simulink model "FSAC2021_V1"  (R2014a)
settings: Solver=FixedStepDiscrete  StartTime=0.0  StopTime=inf  FixedStep=0.0005  RelTol=1e-3
model workspace (MAT data in the model file):
  MCOS : class17 (value not decoded)
  MCOS : class17 (value not decoded)
  MCOS : class17 (value not decoded)
  MCOS : class17 (value not decoded)
  MCOS : class17 (value not decoded)
  MCOS : class17 (value not decoded)
  MCOS : class17 (value not decoded)
  MCOS : class17 (value not decoded)
  MCOS : class17 (value not decoded)
  MCOS : class17 (value not decoded)
  MCOS : class17 (value not decoded)
  MCOS : class17 (value not decoded)
  MCOS : class17 (value not decoded)
  MCOS : class17 (value not decoded)
  MCOS : class17 (value not decoded)
  MCOS : class17 (value not decoded)
  MCOS : class17 (value not decoded)
  MCOS : class17 (value not decoded)
  MCOS : class17 (value not decoded)
  BUZZER_START = 1
  MCOS : class17 (value not decoded)
  MCOS : class17 (value not decoded)
  MCOS : class17 (value not decoded)
  MCOS : class17 (value not decoded)
  MCOS : class17 (value not decoded)
  MCOS : class17 (value not decoded)
  MCOS : class17 (value not decoded)
  MCOS : class17 (value not decoded)
  MCOS : class17 (value not decoded)
  MCOS : class17 (value not decoded)
  MCOS : class17 (value not decoded)
  MCOS : class17 (value not decoded)
  MCOS : class17 (value not decoded)
  MCOS : class17 (value not decoded)
  MCOS : class17 (value not decoded)
  MCOS : class17 (value not decoded)
  MCOS : class17 (value not decoded)
  MCOS : class17 (value not decoded)
  MCOS : class17 (value not decoded)
  MCOS : class17 (value not decoded)
  MCOS : class17 (value not decoded)
  MCOS : class17 (value not decoded)
  MCOS : class17 (value not decoded)
  MCOS : class17 (value not decoded)
  MCOS : class17 (value not decoded)
  MCOS : class17 (value not decoded)
  MCOS : class17 (value not decoded)
  MCOS : class17 (value not decoded)
  MCOS : class17 (value not decoded)
  MCOS : class17 (value not decoded)
  MCOS : class17 (value not decoded)
  MCOS : class17 (value not decoded)
  MCOS : class17 (value not decoded)
  MCOS : class17 (value not decoded)
  MCOS : class17 (value not decoded)
  MCOS : class17 (value not decoded)
  MCOS : class17 (value not decoded)
  MCOS : class17 (value not decoded)
  Brake = 11
  MCOS : class17 (value not decoded)
  MCOS : class17 (value not decoded)
  MCOS : class17 (value not decoded)
  MCOS : class17 (value not decoded)
  MCOS : class17 (value not decoded)
  MCOS : class17 (value not decoded)
  MCOS : class17 (value not decoded)
  MCOS : class17 (value not decoded)
  Sensor_Acc_b = 101.85
  Sensor_Acc_k = -0.0185
  Str_Sen_Orig_Angle = -341
  MCOS : class17 (value not decoded)
  Tire_D = 0.47
  T = 0.05
libraries: simulink x189, ec55xxlib x135
(part 6 of 9)

== system FSAC2021_V1/CAN_SEND/Subsystem1/MOTEC_ENCODER1/Str_Encoder6 ==
  Str_Encoder6 : Inport
  Str_Encoder6Ron : Rounding  Operator=round
  Str_Encoder6_1sat : Saturate  UpperLimit=255  LowerLimit=0
  Str_Encoder6_Convert : DataTypeConversion  OutDataTypeStr=uint8
  Str_Encoder6_Convert1 : DataTypeConversion  OutDataTypeStr=uint32
  Str_Encoder6_D : Product  Inputs=*/
  Str_Encoder6_F : Constant  OutDataTypeStr=single
  Str_Encoder6_L : simulink/Logic and Bit Operations/Bitwise Operator  logicop=AND  UseBitMask=on  BitMask=255  BitMaskRealWorld=Stored Integer
  Str_Encoder6_O : Constant  Value=0  OutDataTypeStr=single
  Str_Encoder6_S : ArithShift
  Str_Encoder6_sat : Saturate  UpperLimit=255  LowerLimit=0
  Str_Encoder6_st : Sum  Inputs=+-
  output6 : Outport
  wires:
  Str_Encoder6/1 -> Str_Encoder6_sat/1
  Str_Encoder6_sat/1 -> Str_Encoder6_st/1
  Str_Encoder6_O/1 -> Str_Encoder6_st/2
  Str_Encoder6_st/1 -> Str_Encoder6_D/1
  Str_Encoder6_F/1 -> Str_Encoder6_D/2
  Str_Encoder6_D/1 -> Str_Encoder6Ron/1
  Str_Encoder6Ron/1 -> Str_Encoder6_S/1
  Str_Encoder6_S/1 -> Str_Encoder6_1sat/1
  Str_Encoder6_1sat/1 -> Str_Encoder6_Convert1/1
  Str_Encoder6_Convert1/1 -> Str_Encoder6_L/1
  Str_Encoder6_L/1 -> Str_Encoder6_Convert/1
  Str_Encoder6_Convert/1 -> output6/1

== system FSAC2021_V1/CAN_SEND/Subsystem1/MOTEC_NMT/NMT_nodectrl ==
  NMT_nodectrl : Inport
  NMT_nodectrlRon : Rounding  Operator=round
  NMT_nodectrl_1sat : Saturate  UpperLimit=255  LowerLimit=0
  NMT_nodectrl_Convert : DataTypeConversion  OutDataTypeStr=uint8
  NMT_nodectrl_Convert1 : DataTypeConversion  OutDataTypeStr=uint32
  NMT_nodectrl_D : Product  Inputs=*/
  NMT_nodectrl_F : Constant  OutDataTypeStr=single
  NMT_nodectrl_L : simulink/Logic and Bit Operations/Bitwise Operator  logicop=AND  UseBitMask=on  BitMask=255  BitMaskRealWorld=Stored Integer
  NMT_nodectrl_O : Constant  Value=0  OutDataTypeStr=single
  NMT_nodectrl_S : ArithShift
  NMT_nodectrl_sat : Saturate  UpperLimit=255  LowerLimit=0
  NMT_nodectrl_st : Sum  Inputs=+-
  output2 : Outport
  wires:
  NMT_nodectrl/1 -> NMT_nodectrl_sat/1
  NMT_nodectrl_sat/1 -> NMT_nodectrl_st/1
  NMT_nodectrl_O/1 -> NMT_nodectrl_st/2
  NMT_nodectrl_st/1 -> NMT_nodectrl_D/1
  NMT_nodectrl_F/1 -> NMT_nodectrl_D/2
  NMT_nodectrl_D/1 -> NMT_nodectrlRon/1
  NMT_nodectrlRon/1 -> NMT_nodectrl_S/1
  NMT_nodectrl_S/1 -> NMT_nodectrl_1sat/1
  NMT_nodectrl_1sat/1 -> NMT_nodectrl_Convert1/1
  NMT_nodectrl_Convert1/1 -> NMT_nodectrl_L/1
  NMT_nodectrl_L/1 -> NMT_nodectrl_Convert/1
  NMT_nodectrl_Convert/1 -> output2/1

== system FSAC2021_V1/CAN_SEND/Subsystem1/MOTEC_NMT/NMT_nodeorder ==
  NMT_nodeorder : Inport
  NMT_nodeorderRon : Rounding  Operator=round
  NMT_nodeorder_1sat : Saturate  UpperLimit=255  LowerLimit=0
  NMT_nodeorder_Convert : DataTypeConversion  OutDataTypeStr=uint8
  NMT_nodeorder_Convert1 : DataTypeConversion  OutDataTypeStr=uint32
  NMT_nodeorder_D : Product  Inputs=*/
  NMT_nodeorder_F : Constant  OutDataTypeStr=single
  NMT_nodeorder_L : simulink/Logic and Bit Operations/Bitwise Operator  logicop=AND  UseBitMask=on  BitMask=255  BitMaskRealWorld=Stored Integer
  NMT_nodeorder_O : Constant  Value=0  OutDataTypeStr=single
  NMT_nodeorder_S : ArithShift
  NMT_nodeorder_sat : Saturate  UpperLimit=255  LowerLimit=0
  NMT_nodeorder_st : Sum  Inputs=+-
  output1 : Outport
  wires:
  NMT_nodeorder/1 -> NMT_nodeorder_sat/1
  NMT_nodeorder_sat/1 -> NMT_nodeorder_st/1
  NMT_nodeorder_O/1 -> NMT_nodeorder_st/2
  NMT_nodeorder_st/1 -> NMT_nodeorder_D/1
  NMT_nodeorder_F/1 -> NMT_nodeorder_D/2
  NMT_nodeorder_D/1 -> NMT_nodeorderRon/1
  NMT_nodeorderRon/1 -> NMT_nodeorder_S/1
  NMT_nodeorder_S/1 -> NMT_nodeorder_1sat/1
  NMT_nodeorder_1sat/1 -> NMT_nodeorder_Convert1/1
  NMT_nodeorder_Convert1/1 -> NMT_nodeorder_L/1
  NMT_nodeorder_L/1 -> NMT_nodeorder_Convert/1
  NMT_nodeorder_Convert/1 -> output1/1

== system FSAC2021_V1/CAN_SEND/Subsystem2/BCU_MTR_MOVE_AB/Brake_mtr_goalpos ==
  Brake_mtr_goalpos : Inport
  Brake_mtr_goalposABS : Abs
  Brake_mtr_goalposBitCov : DataTypeConversion  OutDataTypeStr=uint32
  Brake_mtr_goalposBitCov1 : DataTypeConversion  OutDataTypeStr=uint32
  Brake_mtr_goalposBitCov2 : DataTypeConversion  OutDataTypeStr=uint8
  Brake_mtr_goalposCOV : DataTypeConversion  OutDataTypeStr=uint8
  Brake_mtr_goalposCOV1 : DataTypeConversion  OutDataTypeStr=uint8
  Brake_mtr_goalposCOV2 : DataTypeConversion  OutDataTypeStr=uint8
  Brake_mtr_goalposCS : ArithShift  BitShiftNumber=-32
  Brake_mtr_goalposConS : Constant  OutDataTypeStr=single
  Brake_mtr_goalposCosR : Constant  Value=0  OutDataTypeStr=uint8
  Brake_mtr_goalposROP : RelationalOperator  Operator=<  OutDataTypeStr=boolean
  Brake_mtr_goalposRon : Rounding  Operator=round
  Brake_mtr_goalposSW : Switch  Criteria=u2 ~= 0
  Brake_mtr_goalpos_1sat : Saturate  UpperLimit=4294967295  LowerLimit=0
  Brake_mtr_goalpos_And : simulink/Logic and Bit Operations/Bitwise Operator  logicop=AND  UseBitMask=off  NumInputPorts=2  BitMask=bin2dec('11011001')  BitMaskRealWorld=Stored Integer
  Brake_mtr_goalpos_And1 : simulink/Logic and Bit Operations/Bitwise Operator  logicop=AND  UseBitMask=off  NumInputPorts=2  BitMask=bin2dec('11011001')  BitMaskRealWorld=Stored Integer
  Brake_mtr_goalpos_And1_C : Constant  Value=65535
  Brake_mtr_goalpos_And2 : simulink/Logic and Bit Operations/Bitwise Operator  logicop=AND  UseBitMask=off  NumInputPorts=2  BitMask=bin2dec('11011001')  BitMaskRealWorld=Stored Integer
  Brake_mtr_goalpos_And2_C : Constant  Value=255  OutDataTypeStr=uint32
  Brake_mtr_goalpos_And_C : Constant  Value=16777215
  Brake_mtr_goalpos_Convert : DataTypeConversion  OutDataTypeStr=uint32
  Brake_mtr_goalpos_D{,1..3} (4 alike) : Product  Inputs=*/
  Brake_mtr_goalpos_F : Constant  OutDataTypeStr=single
  Brake_mtr_goalpos_L : simulink/Logic and Bit Operations/Bitwise Operator  logicop=AND  UseBitMask=on  BitMask=4294967295  BitMaskRealWorld=Stored Integer
  Brake_mtr_goalpos_O : Constant  Value=0  OutDataTypeStr=single
  Brake_mtr_goalpos_S : ArithShift
  Brake_mtr_goalpos_sat : Saturate  UpperLimit=2147483647  LowerLimit=-2147483648
  Brake_mtr_goalpos_st : Sum  Inputs=+-
  Brake_mtr_goalpos_swtsig : Switch  Criteria=u2 ~= 0
  Brake_mtr_goalposoutput2_C : Constant  Value=256
  Brake_mtr_goalposoutput3_C : Constant  Value=65536
  Brake_mtr_goalposoutput4_C : Constant  Value=16777216
  Brake_mtr_goalpossatAbs : Saturate  UpperLimit=2147483647  LowerLimit=0
  Brake_mtr_goalpossubcon : Sum  Inputs=+-
  output1 : Outport
  output2 : Outport  Port=2
  output3 : Outport  Port=3
  output4 : Outport  Port=4
  wires:
  Brake_mtr_goalpos/1 -> Brake_mtr_goalpos_sat/1
  Brake_mtr_goalpos_sat/1 -> Brake_mtr_goalpos_st/1
  Brake_mtr_goalpos_O/1 -> Brake_mtr_goalpos_st/2
  Brake_mtr_goalpos_st/1 -> Brake_mtr_goalpos_D/1
  Brake_mtr_goalpos_F/1 -> Brake_mtr_goalpos_D/2
  Brake_mtr_goalpos_D/1 -> Brake_mtr_goalposRon/1
  Brake_mtr_goalpossatAbs/1 -> Brake_mtr_goalpos_swtsig/1, Brake_mtr_goalposSW/3
  Brake_mtr_goalposROP/1 -> Brake_mtr_goalpos_swtsig/2, Brake_mtr_goalposSW/2
  Brake_mtr_goalposRon/1 -> Brake_mtr_goalposROP/1, Brake_mtr_goalposABS/1, Brake_mtr_goalpos_swtsig/3
  Brake_mtr_goalpos_swtsig/1 -> Brake_mtr_goalpossubcon/2
  Brake_mtr_goalposCosR/1 -> Brake_mtr_goalposROP/2
  Brake_mtr_goalposConS/1 -> Brake_mtr_goalposCS/1
  Brake_mtr_goalposCS/1 -> Brake_mtr_goalpossubcon/1
  Brake_mtr_goalposABS/1 -> Brake_mtr_goalpossatAbs/1
  Brake_mtr_goalpossubcon/1 -> Brake_mtr_goalposSW/1
  Brake_mtr_goalposSW/1 -> Brake_mtr_goalpos_S/1
  Brake_mtr_goalpos_S/1 -> Brake_mtr_goalpos_1sat/1
  Brake_mtr_goalpos_1sat/1 -> Brake_mtr_goalpos_Convert/1
  Brake_mtr_goalpos_Convert/1 -> Brake_mtr_goalpos_L/1
  Brake_mtr_goalpos_L/1 -> Brake_mtr_goalpos_And1/1, Brake_mtr_goalpos_And2/1, Brake_mtr_goalpos_And/1, Brake_mtr_goalpos_D1/1
  Brake_mtr_goalposoutput4_C/1 -> Brake_mtr_goalpos_D1/2
  Brake_mtr_goalpos_D1/1 -> Brake_mtr_goalposCOV/1
  Brake_mtr_goalposCOV/1 -> output1/1
  Brake_mtr_goalpos_And_C/1 -> Brake_mtr_goalposBitCov/1
  Brake_mtr_goalposBitCov/1 -> Brake_mtr_goalpos_And/2
  Brake_mtr_goalpos_And/1 -> Brake_mtr_goalpos_D2/1
  Brake_mtr_goalposoutput3_C/1 -> Brake_mtr_goalpos_D2/2
  Brake_mtr_goalpos_D2/1 -> Brake_mtr_goalposCOV1/1
  Brake_mtr_goalposCOV1/1 -> output2/1
  Brake_mtr_goalpos_And1_C/1 -> Brake_mtr_goalposBitCov1/1
  Brake_mtr_goalposBitCov1/1 -> Brake_mtr_goalpos_And1/2
  Brake_mtr_goalpos_And1/1 -> Brake_mtr_goalpos_D3/1
  Brake_mtr_goalposoutput2_C/1 -> Brake_mtr_goalpos_D3/2
  Brake_mtr_goalpos_D3/1 -> Brake_mtr_goalposCOV2/1
  Brake_mtr_goalposCOV2/1 -> output3/1
  Brake_mtr_goalpos_And2_C/1 -> Brake_mtr_goalpos_And2/2
  Brake_mtr_goalpos_And2/1 -> Brake_mtr_goalposBitCov2/1
  Brake_mtr_goalposBitCov2/1 -> output4/1

== system FSAC2021_V1/CAN_SEND/Subsystem2/MOTOR_SPEED_CONTROL/Drive_Speed_Control ==
  Drive_Speed_Control : Inport
  BitCov : DataTypeConversion  OutDataTypeStr=uint8
  Drive_Speed_ControlCOV : DataTypeConversion  OutDataTypeStr=uint8
  Drive_Speed_ControlRon : Rounding  Operator=round
  Drive_Speed_Control_1sat : Saturate  UpperLimit=65535  LowerLimit=0
  Drive_Speed_Control_And : simulink/Logic and Bit Operations/Bitwise Operator  logicop=AND  UseBitMask=off  NumInputPorts=2  BitMask=bin2dec('11011001')  BitMaskRealWorld=Stored Integer
  Drive_Speed_Control_And_C : Constant  Value=255  OutDataTypeStr=uint32
  Drive_Speed_Control_Convert : DataTypeConversion  OutDataTypeStr=uint32
  Drive_Speed_Control_D : Product  Inputs=*/
  Drive_Speed_Control_D1 : Product  Inputs=*/
  Drive_Speed_Control_F : Constant  OutDataTypeStr=single
  Drive_Speed_Control_L : simulink/Logic and Bit Operations/Bitwise Operator  logicop=AND  UseBitMask=on  BitMask=65535  BitMaskRealWorld=Stored Integer
  Drive_Speed_Control_O : Constant  Value=0  OutDataTypeStr=single
  Drive_Speed_Control_S : ArithShift
  Drive_Speed_Control_sat : Saturate  UpperLimit=1500  LowerLimit=0
  Drive_Speed_Control_st : Sum  Inputs=+-
  Drive_Speed_Controloutput2_C : Constant  Value=256
  output1 : Outport
  output2 : Outport  Port=2
  wires:
  Drive_Speed_Control/1 -> Drive_Speed_Control_sat/1
  Drive_Speed_Control_sat/1 -> Drive_Speed_Control_st/1
  Drive_Speed_Control_O/1 -> Drive_Speed_Control_st/2
  Drive_Speed_Control_st/1 -> Drive_Speed_Control_D/1
  Drive_Speed_Control_F/1 -> Drive_Speed_Control_D/2
  Drive_Speed_Control_D/1 -> Drive_Speed_ControlRon/1
  Drive_Speed_ControlRon/1 -> Drive_Speed_Control_S/1
  Drive_Speed_Control_S/1 -> Drive_Speed_Control_1sat/1
  Drive_Speed_Control_1sat/1 -> Drive_Speed_Control_Convert/1
  Drive_Speed_Control_Convert/1 -> Drive_Speed_Control_L/1
  Drive_Speed_Control_L/1 -> Drive_Speed_Control_D1/1, Drive_Speed_Control_And/1
  Drive_Speed_Controloutput2_C/1 -> Drive_Speed_Control_D1/2
  Drive_Speed_Control_D1/1 -> Drive_Speed_ControlCOV/1
  Drive_Speed_ControlCOV/1 -> output2/1
  Drive_Speed_Control_And_C/1 -> Drive_Speed_Control_And/2
  Drive_Speed_Control_And/1 -> BitCov/1
  BitCov/1 -> output1/1

== system FSAC2021_V1/CAN_SEND/Subsystem3/BCU_STATUS_READ/status_reg_addr_start ==
  status_reg_addr_start : Inport
  status_reg_addr_startRon : Rounding  Operator=round
  status_reg_addr_start_1sat : Saturate  UpperLimit=255  LowerLimit=0
  status_reg_addr_start_Convert : DataTypeConversion  OutDataTypeStr=uint8
  status_reg_addr_start_Convert1 : DataTypeConversion  OutDataTypeStr=uint32
  status_reg_addr_start_D : Product  Inputs=*/
  status_reg_addr_start_F : Constant  OutDataTypeStr=single
  status_reg_addr_start_L : simulink/Logic and Bit Operations/Bitwise Operator  logicop=AND  UseBitMask=on  BitMask=255  BitMaskRealWorld=Stored Integer
  status_reg_addr_start_O : Constant  Value=0  OutDataTypeStr=single
  status_reg_addr_start_S : ArithShift
  status_reg_addr_start_sat : Saturate  UpperLimit=255  LowerLimit=0
  status_reg_addr_start_st : Sum  Inputs=+-
  output1 : Outport
  wires:
  status_reg_addr_start/1 -> status_reg_addr_start_sat/1
  status_reg_addr_start_sat/1 -> status_reg_addr_start_st/1
  status_reg_addr_start_O/1 -> status_reg_addr_start_st/2
  status_reg_addr_start_st/1 -> status_reg_addr_start_D/1
  status_reg_addr_start_F/1 -> status_reg_addr_start_D/2
  status_reg_addr_start_D/1 -> status_reg_addr_startRon/1
  status_reg_addr_startRon/1 -> status_reg_addr_start_S/1
  status_reg_addr_start_S/1 -> status_reg_addr_start_1sat/1
  status_reg_addr_start_1sat/1 -> status_reg_addr_start_Convert1/1
  status_reg_addr_start_Convert1/1 -> status_reg_addr_start_L/1
  status_reg_addr_start_L/1 -> status_reg_addr_start_Convert/1
  status_reg_addr_start_Convert/1 -> output1/1

== system FSAC2021_V1/CAN_SEND/Subsystem3/BCU_STATUS_READ/status_reg_num ==
  status_reg_num : Inport
  status_reg_numRon : Rounding  Operator=round
  status_reg_num_1sat : Saturate  UpperLimit=255  LowerLimit=0
  status_reg_num_Convert : DataTypeConversion  OutDataTypeStr=uint8
  status_reg_num_Convert1 : DataTypeConversion  OutDataTypeStr=uint32
  status_reg_num_D : Product  Inputs=*/
  status_reg_num_F : Constant  OutDataTypeStr=single
  status_reg_num_L : simulink/Logic and Bit Operations/Bitwise Operator  logicop=AND  UseBitMask=on  BitMask=255  BitMaskRealWorld=Stored Integer
  status_reg_num_O : Constant  Value=0  OutDataTypeStr=single
  status_reg_num_S : ArithShift
  status_reg_num_sat : Saturate  UpperLimit=255  LowerLimit=0
  status_reg_num_st : Sum  Inputs=+-
  output2 : Outport
  wires:
  status_reg_num/1 -> status_reg_num_sat/1
  status_reg_num_sat/1 -> status_reg_num_st/1
  status_reg_num_O/1 -> status_reg_num_st/2
  status_reg_num_st/1 -> status_reg_num_D/1
  status_reg_num_F/1 -> status_reg_num_D/2
  status_reg_num_D/1 -> status_reg_numRon/1
  status_reg_numRon/1 -> status_reg_num_S/1
  status_reg_num_S/1 -> status_reg_num_1sat/1
  status_reg_num_1sat/1 -> status_reg_num_Convert1/1
  status_reg_num_Convert1/1 -> status_reg_num_L/1
  status_reg_num_L/1 -> status_reg_num_Convert/1
  status_reg_num_Convert/1 -> output2/1

== system FSAC2021_V1/Controller/200ms_Duty/Light_Subsystem/BLINK  ==
  Action Port : ActionPort  ActionType=else
  Data Type Conversion : DataTypeConversion  OutDataTypeStr=uint8
  Logical Operator : Logic  Operator=NOT  AllPortsSameDT=off  OutDataTypeStr=boolean
  Unit Delay : UnitDelay  SampleTime=-1
  Out1 : Outport
  wires:
  Logical Operator/1 -> Data Type Conversion/1
  Data Type Conversion/1 -> Unit Delay/1, Out1/1
  Unit Delay/1 -> Logical Operator/1

== system FSAC2021_V1/Controller/200ms_Duty/Light_Subsystem/OFF ==
  Action Port : ActionPort  ActionType=elseif
  Constant : Constant  OutDataTypeStr=uint8
  Out1 : Outport
  wires:
  Constant/1 -> Out1/1

== system FSAC2021_V1/Controller/200ms_Duty/Light_Subsystem/ON ==
  Action Port : ActionPort  ActionType=then
  Constant : Constant  Value=0  OutDataTypeStr=uint8
  Out1 : Outport
  wires:
  Constant/1 -> Out1/1

== system FSAC2021_V1/Controller/200ms_Duty/Light_Subsystem1/BLINK ==
  Action Port : ActionPort  ActionType=else
  Data Type Conversion : DataTypeConversion  OutDataTypeStr=uint8
  Logical Operator : Logic  Operator=NOT  AllPortsSameDT=off  OutDataTypeStr=boolean
  Unit Delay : UnitDelay  SampleTime=-1
  Out1 : Outport
  wires:
  Unit Delay/1 -> Logical Operator/1
  Data Type Conversion/1 -> Out1/1, Unit Delay/1
  Logical Operator/1 -> Data Type Conversion/1

== system FSAC2021_V1/Controller/200ms_Duty/Light_Subsystem1/OFF ==
  Action Port : ActionPort  ActionType=elseif
  Constant : Constant  OutDataTypeStr=uint8
  Out1 : Outport
  wires:
  Constant/1 -> Out1/1

== system FSAC2021_V1/Controller/200ms_Duty/Light_Subsystem1/ON ==
  Action Port : ActionPort  ActionType=then
  Constant : Constant  Value=0  OutDataTypeStr=uint8
  Out1 : Outport
  wires:
  Constant/1 -> Out1/1

== system FSAC2021_V1/Controller/200ms_Duty/Light_Subsystem2/EBS_Horn ==
  Action Port : ActionPort  ActionType=else
  Chart : Stateflow chart  TreatAsAtomicUnit=on
  Buzzer_Pin : Outport
  Buzzer_Overflag : Outport  Port=2
  wires:
  Chart/1(Buzzer_Pin) -> Buzzer_Pin/1
  Chart/2(Buzzer_Overflag) -> Buzzer_Overflag/1

== system FSAC2021_V1/Controller/200ms_Duty/Light_Subsystem2/Start_Horn ==
  Action Port : ActionPort  ActionType=elseif
  Chart : Stateflow chart  TreatAsAtomicUnit=on
  Out1 : Outport
  wires:
  Chart/1(Buzzer_Pin) -> Out1/1

== system FSAC2021_V1/Controller/200ms_Duty/Light_Subsystem2/off ==
  Action Port : ActionPort  ActionType=then
  Constant : Constant  Value=0  OutDataTypeStr=uint8
  Out1 : Outport
  wires:
  Constant/1 -> Out1/1

== system FSAC2021_V1/Controller/50ms_Duty/Subsystem/Subsystem ==
  acc : Inport
  Acc_Flag : Inport  Port=2
  Enable : EnablePort
  Constant : Constant  Value=0
  Switch : Switch  Criteria=u2 > Threshold
  Acc_Cmd : Outport
  wires:
  Acc_Flag/1 -> Switch/2
  Constant/1 -> Switch/1
  acc/1 -> Switch/3
  Switch/1 -> Acc_Cmd/1

== system FSAC2021_V1/Controller/50ms_Duty/Subsystem/Subsystem1 ==
  IPC_Acc_Cmd : Inport
  IPC_Brk_Cmd : Inport  Port=2
  IPC_Str_Cmd : Inport  Port=3
  Enable : EnablePort
  Data Type Conversion : DataTypeConversion
  Gain : Gain  Gain=15
  Gain1 : Gain  Gain=0.134
  Saturation : Saturate  UpperLimit=13.4  LowerLimit=0
  Brk_Cmd : Outport
  Str_Cmd : Outport  Port=2
  Acc_Cmd : Outport  Port=3
  wires:
  IPC_Str_Cmd/1 -> Str_Cmd/1
  Gain/1 -> Acc_Cmd/1
  IPC_Brk_Cmd/1 -> Gain1/1
  Gain1/1 -> Saturation/1
  Saturation/1 -> Data Type Conversion/1
  IPC_Acc_Cmd/1 -> Gain/1
  Data Type Conversion/1 -> Brk_Cmd/1

== system FSAC2021_V1/Controller/50ms_Duty/Subsystem/Subsystem2 ==
  Enable : EnablePort
  Chart : Stateflow chart  TreatAsAtomicUnit=on
  ACC : Outport
  SteerCmd : Outport  Port=2
  Mission_Flag : Outport  Port=3
  wires:
  Chart/1(Mission_Flag) -> Mission_Flag/1
  Chart/3(ACC) -> ACC/1
  Chart/2(SteerCmd) -> SteerCmd/1

== system FSAC2021_V1/Controller/BCU_Controller/Brk_Move/Enabled Subsystem ==
  Enable : EnablePort
  Angle2Pulses : Subsystem  TreatAsAtomicUnit=on
  Constant : Constant  Value=BRK_Engaged_Angle  OutDataTypeStr=int8
  Engaged_Pulses : Outport
  Engaged_Angle : Outport  Port=2
  wires:
  Angle2Pulses/1(Pulses) -> Engaged_Pulses/1
  Constant/1 -> Angle2Pulses/1(Angle), Engaged_Angle/1

== system FSAC2021_V1/Controller/BCU_Controller/Brk_Move/Enabled Subsystem1 ==
  Engaged_Angle : Inport
  Enable : EnablePort
  Angle2Pulses : Subsystem  TreatAsAtomicUnit=on
  Gain : Gain  ParamDataTypeStr=int8  OutDataTypeStr=int8
  ToZero_Pulses : Outport
  wires:
  Angle2Pulses/1(Pulses) -> ToZero_Pulses/1
  Engaged_Angle/1 -> Gain/1
  Gain/1 -> Angle2Pulses/1(Angle)

== system FSAC2021_V1/Controller/BCU_Controller/Brk_Move/Enabled Subsystem2 ==
  note: 制动百分比
  note: 电机反转
  Brk_Prop : Inport
  Enable : EnablePort
  Angle2Pulses : Subsystem  TreatAsAtomicUnit=on
  Brk_Prop2Angle : Gain  Gain=Brk_Prop2Angle
  Gain : Gain  Gain=-1  ParamDataTypeStr=int8  OutDataTypeStr=single
  Move_Pulses : Outport
  wires:
  Gain/1 -> Angle2Pulses/1(Angle)
  Brk_Prop/1 -> Brk_Prop2Angle/1
  Brk_Prop2Angle/1 -> Gain/1
  Angle2Pulses/1(Pulses) -> Move_Pulses/1

== system FSAC2021_V1/DIAG/DIAG/ACC/Enabled Subsystem ==
  liquid_presuress : Inport
  Acc_Ctrl : Inport  Port=2
  Enable : EnablePort
  Chart : Stateflow chart  TreatAsAtomicUnit=on
  Acc_Flag : Outport
  wires:
  liquid_presuress/1 -> Chart/1(liquid_presuress)
  Acc_Ctrl/1 -> Chart/2(Acc)
  Chart/1(Acc_Flag) -> Acc_Flag/1

== system FSAC2021_V1/DIAG/DIAG/CAN_NODE_LOSTCOM/B_M_S_Check ==
  Brake_Node : Inport
  Motec_Node : Inport  Port=2
  RES_Node : Inport  Port=3
  Enable : EnablePort
  Chart : Stateflow chart  TreatAsAtomicUnit=on
      settings: RTWSystemCode=Reusable function
  Chart1 : Stateflow chart  TreatAsAtomicUnit=on
      settings: RTWSystemCode=Reusable function
  Logical Operator : Logic  AllPortsSameDT=off  OutDataTypeStr=boolean
  MeaModule1 : ec55xxlib/RapidECU_U2/11Calibration/MeaModule  signal=BRAKE
  MeaModule2 : ec55xxlib/RapidECU_U2/11Calibration/MeaModule  signal=MOTEC
  Node_Lost_Flag : Outport
  wires:
  Logical Operator/1 -> Node_Lost_Flag/1
  Brake_Node/1 -> Chart1/1(Input)
  MeaModule1/1 -> Logical Operator/1
  MeaModule2/1 -> Logical Operator/2
  Motec_Node/1 -> Chart/1(Input)
  Chart/1(Output) -> MeaModule2/1
  Chart1/1(Output) -> MeaModule1/1

== system FSAC2021_V1/DIAG/DIAG/CAN_NODE_LOSTCOM/Subsystem ==
  Motor_Node : Inport
  Enable : EnablePort
  Chart4 : Stateflow chart  TreatAsAtomicUnit=on
      settings: RTWSystemCode=Reusable function
  MeaModule1 : ec55xxlib/RapidECU_U2/11Calibration/MeaModule  signal=motor
  Node_Lost_Flag : Outport
  wires:
  MeaModule1/1 -> Node_Lost_Flag/1
  Motor_Node/1 -> Chart4/1(Input)
  Chart4/1(Output) -> MeaModule1/1

== system FSAC2021_V1/DIAG/DIAG/CAN_NODE_LOSTCOM/Subsystem1 ==
  StrSr_Node : Inport
  BMS_Node : Inport  Port=2
  AMI_Node : Inport  Port=3
  Chart2 : Stateflow chart  TreatAsAtomicUnit=on
      settings: RTWSystemCode=Reusable function
  Chart3 : Stateflow chart  TreatAsAtomicUnit=on
      settings: RTWSystemCode=Reusable function
  Chart4 : Stateflow chart  TreatAsAtomicUnit=on
      settings: RTWSystemCode=Reusable function
  Logical Operator : Logic  Inputs=3  AllPortsSameDT=off  OutDataTypeStr=boolean
  MeaModule3 : ec55xxlib/RapidECU_U2/11Calibration/MeaModule  signal=STRSNR
  MeaModule4 : ec55xxlib/RapidECU_U2/11Calibration/MeaModule  signal=BMS
  MeaModule5 : ec55xxlib/RapidECU_U2/11Calibration/MeaModule  signal=AMI_NODE
  Out1 : Outport
  wires:
  StrSr_Node/1 -> Chart2/1(Input)
  Chart2/1(Output) -> MeaModule3/1
  Chart4/1(Output) -> MeaModule5/1
  Chart3/1(Output) -> MeaModule4/1
  BMS_Node/1 -> Chart3/1(Input)
  AMI_Node/1 -> Chart4/1(Input)
  MeaModule3/1 -> Logical Operator/1
  MeaModule4/1 -> Logical Operator/2
  MeaModule5/1 -> Logical Operator/3
  Logical Operator/1 -> Out1/1

== system FSAC2021_V1/DIAG/DIAG/Res_Diag/Subsystem ==
  RES_SINGNAL : Inport
  Enable : EnablePort
  Chart1 : Stateflow chart  TreatAsAtomicUnit=on
      settings: RTWSystemCode=Reusable function
  Compare To Constant1 : simulink/Logic and Bit Operations/Compare To Constant  relop===  const=8  OutDataTypeStr=boolean
  Compare To Constant2 : simulink/Logic and Bit Operations/Compare To Constant  relop===  const=0  OutDataTypeStr=boolean
  Data Type Conversion1 : DataTypeConversion
  Data Type Conversion22 : DataTypeConversion
  Data Type Conversion23 : DataTypeConversion
  MeaModule1 : ec55xxlib/RapidECU_U2/11Calibration/MeaModule  signal=res_ebs_value
  RES_GO : Outport
  RES_EBS : Outport  Port=2
  wires:
  Compare To Constant1/1 -> Data Type Conversion22/1
  Data Type Conversion22/1 -> RES_GO/1
  Data Type Conversion23/1 -> MeaModule1/1
  RES_SINGNAL/1 -> Compare To Constant2/1, Compare To Constant1/1
  MeaModule1/1 -> RES_EBS/1
  Chart1/1(Output) -> Data Type Conversion23/1
  Compare To Constant2/1 -> Data Type Conversion1/1
  Data Type Conversion1/1 -> Chart1/1(Input)

== system FSAC2021_V1/DIAG/DIAG/TS_Diag/Subsystem ==
  Compare_Volt_mv : Inport
  Enable : EnablePort
  Compare To Constant3 : simulink/Logic and Bit Operations/Compare To Constant  relop=<  const=2  OutDataTypeStr=boolean
  TS_Error : Outport
  wires:
  Compare_Volt_mv/1 -> Compare To Constant3/1
  Compare To Constant3/1 -> TS_Error/1

== system FSAC2021_V1/DIAG/DIAG/TS_Diag/Subsystem1 ==
  Compare_Volt_mv : Inport
  Enable : EnablePort
  Compare To Constant3 : simulink/Logic and Bit Operations/Compare To Constant  relop=<  const=2  OutDataTypeStr=boolean
  TS_Error : Outport
  wires:
  Compare_Volt_mv/1 -> Compare To Constant3/1
  Compare To Constant3/1 -> TS_Error/1

== system FSAC2021_V1/DIAG/DIAG/TS_Diag/Subsystem2 ==
  Compare_Volt_mv : Inport
  Enable : EnablePort
  Compare To Constant3 : simulink/Logic and Bit Operations/Compare To Constant  relop=<  const=2  OutDataTypeStr=boolean
  TS_Error : Outport
  wires:
  Compare_Volt_mv/1 -> Compare To Constant3/1
  Compare To Constant3/1 -> TS_Error/1

== system FSAC2021_V1/Input_Process/KL_Sig_Process/Whl_Spd_Process/LPF ==
  note: y(t) = K*u(t) + (1-K)*y(t-1) = y(t-1) + K*[u(t)-y(t-1)]
      | 其中，K=dT/T，K一般介于0~1之间，dT是运行步长，T是时间常数；u是输入信号；y是输出信号。
  Filter : Inport
  Add : Sum  Inputs=+-  AccumDataTypeStr=single
  Add1 : Sum  AccumDataTypeStr=single
  Constant : Constant  Value=Filter_Factor
  Product : Product  OutDataTypeStr=single
  Unit Delay : UnitDelay  InitialCondition=1  SampleTime=-1
  Filtered : Outport
  wires:
  Add1/1 -> Unit Delay/1, Filtered/1
  Filter/1 -> Add/1
  Unit Delay/1 -> Add1/2, Add/2
  Add/1 -> Product/2
  Constant/1 -> Product/1
  Product/1 -> Add1/1

== system FSAC2021_V1/Input_Process/KL_Sig_Process/Whl_Spd_Process/LPF1 ==
  note: y(t) = K*u(t) + (1-K)*y(t-1) = y(t-1) + K*[u(t)-y(t-1)]
      | 其中，K=dT/T，K一般介于0~1之间，dT是运行步长，T是时间常数；u是输入信号；y是输出信号。
  Filter : Inport
  Add : Sum  Inputs=+-  AccumDataTypeStr=single
  Add1 : Sum  AccumDataTypeStr=single
  Constant : Constant  Value=Filter_Factor
  Product : Product  OutDataTypeStr=single
  Unit Delay : UnitDelay  InitialCondition=1  SampleTime=-1
  Filtered : Outport
  wires:
  Product/1 -> Add1/1
  Constant/1 -> Product/1
  Add/1 -> Product/2
  Unit Delay/1 -> Add/2, Add1/2
  Filter/1 -> Add/1
  Add1/1 -> Filtered/1, Unit Delay/1

== system FSAC2021_V1/Input_Process/KL_Sig_Process/Whl_Spd_Process/LPF2 ==
  note: y(t) = K*u(t) + (1-K)*y(t-1) = y(t-1) + K*[u(t)-y(t-1)]
      | 其中，K=dT/T，K一般介于0~1之间，dT是运行步长，T是时间常数；u是输入信号；y是输出信号。
  Filter : Inport
  Add : Sum  Inputs=+-  AccumDataTypeStr=single
  Add1 : Sum  AccumDataTypeStr=single
  Constant : Constant  Value=Filter_Factor
  Product : Product  OutDataTypeStr=single
  Unit Delay : UnitDelay  InitialCondition=1  SampleTime=-1
  Filtered : Outport
  wires:
  Add1/1 -> Unit Delay/1, Filtered/1
  Filter/1 -> Add/1
  Unit Delay/1 -> Add1/2, Add/2
  Add/1 -> Product/2
  Constant/1 -> Product/1
  Product/1 -> Add1/1

== system FSAC2021_V1/Input_Process/KL_Sig_Process/Whl_Spd_Process/LPF3 ==
  note: y(t) = K*u(t) + (1-K)*y(t-1) = y(t-1) + K*[u(t)-y(t-1)]
      | 其中，K=dT/T，K一般介于0~1之间，dT是运行步长，T是时间常数；u是输入信号；y是输出信号。
  Filter : Inport
  Add : Sum  Inputs=+-  AccumDataTypeStr=single
  Add1 : Sum  AccumDataTypeStr=single
  Constant : Constant  Value=Filter_Factor
  Product : Product  OutDataTypeStr=single
  Unit Delay : UnitDelay  InitialCondition=1  SampleTime=-1
  Filtered : Outport
  wires:
  Product/1 -> Add1/1
  Constant/1 -> Product/1
  Add/1 -> Product/2
  Unit Delay/1 -> Add/2, Add1/2
  Filter/1 -> Add/1
  Add1/1 -> Filtered/1, Unit Delay/1

== system FSAC2021_V1/Input_Process/KL_Sig_Process/Whl_Spd_Process/Whl2Veh_Spd_Trans ==
  Wheel_speed_rightrear_wheel : Inport
  Wheel_speed_right_front_wheel : Inport  Port=2
  Wheel_speed_leftrear_wheel : Inport  Port=3
  Wheel_speed_leftfront_wheel : Inport  Port=4
  Round : Subsystem  TreatAsAtomicUnit=on
  Wheel_Mean : Subsystem
  rpm2km_h : Subsystem
  Vel_Speed : Outport
  wires:
  Wheel_speed_leftfront_wheel/1 -> Wheel_Mean/4(Wheel_speed_leftfront_wheel)
  Wheel_speed_leftrear_wheel/1 -> Wheel_Mean/3(Wheel_speed_leftrear_wheel)
  Wheel_speed_rightrear_wheel/1 -> Wheel_Mean/1(Wheel_speed_rightrear_wheel)
  Wheel_speed_right_front_wheel/1 -> Wheel_Mean/2(Wheel_speed_right_front_wheel)
  Wheel_Mean/1(Out1) -> rpm2km_h/1(rpm)
  rpm2km_h/1(kmph) -> Round/1(Origin_Precision)
  Round/1(Two_Precision) -> Vel_Speed/1

== system FSAC2021_V1/Input_Process/KL_Sig_Process/Whl_Spd_Process/Whl_Spd_Hz2RPM ==
  Whl_Spd_Hz : Inport  OutDataTypeStr=uint32
  Constant : Constant  Value=FTeeth_Wheel  OutDataTypeStr=single
  Divide : Product  Inputs=*/
  rps2rpm : Gain  Gain=60  ParamDataTypeStr=uint16  OutDataTypeStr=single
  Whl_Spd_RPM : Outport
  wires:
  Divide/1 -> rps2rpm/1
  Constant/1 -> Divide/2
  Whl_Spd_Hz/1 -> Divide/1
  rps2rpm/1 -> Whl_Spd_RPM/1

== system FSAC2021_V1/Input_Process/KL_Sig_Process/Whl_Spd_Process/Whl_Spd_Hz2RPM1 ==
  Whl_Spd_Hz : Inport  OutDataTypeStr=uint32
  Constant : Constant  Value=FTeeth_Wheel  OutDataTypeStr=single
  Divide : Product  Inputs=*/
  rps2rpm : Gain  Gain=60  ParamDataTypeStr=uint16  OutDataTypeStr=single
  Whl_Spd_RPM : Outport
  wires:
  rps2rpm/1 -> Whl_Spd_RPM/1
  Whl_Spd_Hz/1 -> Divide/1
  Constant/1 -> Divide/2
  Divide/1 -> rps2rpm/1

== system FSAC2021_V1/Input_Process/KL_Sig_Process/Whl_Spd_Process/Whl_Spd_Hz2RPM2 ==
  Whl_Spd_Hz : Inport  OutDataTypeStr=uint32
  Constant : Constant  Value=RTeeth_Wheel  OutDataTypeStr=single
  Divide : Product  Inputs=*/
  rps2rpm : Gain  Gain=60  ParamDataTypeStr=uint16  OutDataTypeStr=single
  Whl_Spd_RPM : Outport
  wires:
  Divide/1 -> rps2rpm/1
  Constant/1 -> Divide/2
  Whl_Spd_Hz/1 -> Divide/1
  rps2rpm/1 -> Whl_Spd_RPM/1

== system FSAC2021_V1/Input_Process/KL_Sig_Process/Whl_Spd_Process/Whl_Spd_Hz2RPM3 ==
  Whl_Spd_Hz : Inport  OutDataTypeStr=uint32
  Constant : Constant  Value=RTeeth_Wheel  OutDataTypeStr=single
  Divide : Product  Inputs=*/
  rps2rpm : Gain  Gain=60  ParamDataTypeStr=uint16  OutDataTypeStr=single
  Whl_Spd_RPM : Outport
  wires:
  rps2rpm/1 -> Whl_Spd_RPM/1
  Whl_Spd_Hz/1 -> Divide/1
  Constant/1 -> Divide/2
  Divide/1 -> rps2rpm/1

== system FSAC2021_V1/VCU_CAN_Read/PCANA(RES、AMI、MOTEC、BRAKE、STEER_SENSOR、IPC)/BCU_MTR_STATUS1/Brake_cmd_fault_flag_Sub ==
  In1 : Inport
  Out1 : Outport
  wires:
  In1/1 -> Out1/1

== system FSAC2021_V1/VCU_CAN_Read/PCANA(RES、AMI、MOTEC、BRAKE、STEER_SENSOR、IPC)/BCU_MTR_STATUS1/Brake_encoder_fault_sts_Sub ==
  In1 : Inport
  Out1 : Outport
  wires:
  In1/1 -> Out1/1

== system FSAC2021_V1/VCU_CAN_Read/PCANA(RES、AMI、MOTEC、BRAKE、STEER_SENSOR、IPC)/BCU_MTR_STATUS1/Brake_go_origin_over_flag_Sub ==
  In1 : Inport
  Out1 : Outport
  wires:
  In1/1 -> Out1/1

== system FSAC2021_V1/VCU_CAN_Read/PCANA(RES、AMI、MOTEC、BRAKE、STEER_SENSOR、IPC)/BCU_MTR_STATUS1/Brake_hd_fault_sts_Sub ==
  In1 : Inport
  Out1 : Outport
  wires:
  In1/1 -> Out1/1

== system FSAC2021_V1/VCU_CAN_Read/PCANA(RES、AMI、MOTEC、BRAKE、STEER_SENSOR、IPC)/BCU_MTR_STATUS1/Brake_lowvolt_prtct_sts_Sub ==
  In1 : Inport
  Out1 : Outport
  wires:
  In1/1 -> Out1/1

== system FSAC2021_V1/VCU_CAN_Read/PCANA(RES、AMI、MOTEC、BRAKE、STEER_SENSOR、IPC)/BCU_MTR_STATUS1/Brake_mtr_enable_flag_Sub ==
  In1 : Inport
  Out1 : Outport
  wires:
  In1/1 -> Out1/1

== system FSAC2021_V1/VCU_CAN_Read/PCANA(RES、AMI、MOTEC、BRAKE、STEER_SENSOR、IPC)/BCU_MTR_STATUS1/Brake_mtr_goalpos_Sub ==
  In1 : Inport
  Out1 : Outport
  wires:
  In1/1 -> Out1/1

== system FSAC2021_V1/VCU_CAN_Read/PCANA(RES、AMI、MOTEC、BRAKE、STEER_SENSOR、IPC)/BCU_MTR_STATUS1/Brake_mtr_origin_flag_Sub ==
  In1 : Inport
  Out1 : Outport
  wires:
  In1/1 -> Out1/1

== system FSAC2021_V1/VCU_CAN_Read/PCANA(RES、AMI、MOTEC、BRAKE、STEER_SENSOR、IPC)/BCU_MTR_STATUS1/Brake_mtr_stop_flag_Sub ==
  In1 : Inport
  Out1 : Outport
  wires:
  In1/1 -> Out1/1

== system FSAC2021_V1/VCU_CAN_Read/PCANA(RES、AMI、MOTEC、BRAKE、STEER_SENSOR、IPC)/BCU_MTR_STATUS1/Brake_offline_run_flag_Sub ==
  In1 : Inport
  Out1 : Outport
  wires:
  In1/1 -> Out1/1

== system FSAC2021_V1/VCU_CAN_Read/PCANA(RES、AMI、MOTEC、BRAKE、STEER_SENSOR、IPC)/BCU_MTR_STATUS1/Brake_overcurrt_prtct_sts_Sub ==
  In1 : Inport
  Out1 : Outport
  wires:
  In1/1 -> Out1/1

== system FSAC2021_V1/VCU_CAN_Read/PCANA(RES、AMI、MOTEC、BRAKE、STEER_SENSOR、IPC)/BCU_MTR_STATUS1/Brake_overheat_prtct_sts_Sub ==
  In1 : Inport
  Out1 : Outport
  wires:
  In1/1 -> Out1/1

== system FSAC2021_V1/VCU_CAN_Read/PCANA(RES、AMI、MOTEC、BRAKE、STEER_SENSOR、IPC)/BCU_MTR_STATUS1/Brake_pos_enqual_Sub ==
  In1 : Inport
  Out1 : Outport
  wires:
  In1/1 -> Out1/1

== system FSAC2021_V1/VCU_CAN_Read/PCANA(RES、AMI、MOTEC、BRAKE、STEER_SENSOR、IPC)/BCU_MTR_STATUS1/Brake_reg_rw_fault_flag_Sub ==
  In1 : Inport
  Out1 : Outport
  wires:
  In1/1 -> Out1/1

== system FSAC2021_V1/VCU_CAN_Read/PCANA(RES、AMI、MOTEC、BRAKE、STEER_SENSOR、IPC)/BCU_MTR_STATUS1/Brake_sensor1_sts_Sub ==
  In1 : Inport
  Out1 : Outport
  wires:
  In1/1 -> Out1/1

== system FSAC2021_V1/VCU_CAN_Read/PCANA(RES、AMI、MOTEC、BRAKE、STEER_SENSOR、IPC)/BCU_MTR_STATUS1/Brake_sensor2_sts_Sub ==
  In1 : Inport
  Out1 : Outport
  wires:
  In1/1 -> Out1/1

== system FSAC2021_V1/VCU_CAN_Read/PCANA(RES、AMI、MOTEC、BRAKE、STEER_SENSOR、IPC)/BCU_MTR_STATUS1/Brake_sensor3_sts_Sub ==
  In1 : Inport
  Out1 : Outport
  wires:
  In1/1 -> Out1/1

== system FSAC2021_V1/VCU_CAN_Read/PCANA(RES、AMI、MOTEC、BRAKE、STEER_SENSOR、IPC)/BCU_MTR_STATUS1/Brake_sensor4_sts_Sub ==
  In1 : Inport
  Out1 : Outport
  wires:
  In1/1 -> Out1/1

== system FSAC2021_V1/VCU_CAN_Read/PCANA(RES、AMI、MOTEC、BRAKE、STEER_SENSOR、IPC)/BCU_MTR_STATUS1/Brake_sensor5_sts_Sub ==
  In1 : Inport
  Out1 : Outport
  wires:
  In1/1 -> Out1/1

== system FSAC2021_V1/VCU_CAN_Read/PCANA(RES、AMI、MOTEC、BRAKE、STEER_SENSOR、IPC)/BCU_MTR_STATUS1/Brake_sensor6_sts_Sub ==
  In1 : Inport
  Out1 : Outport
  wires:
  In1/1 -> Out1/1

== system FSAC2021_V1/VCU_CAN_Read/PCANA(RES、AMI、MOTEC、BRAKE、STEER_SENSOR、IPC)/BCU_MTR_STATUS1/Brake_speed_enqual_Sub ==
  In1 : Inport
  Out1 : Outport
  wires:
  In1/1 -> Out1/1

== system FSAC2021_V1/VCU_CAN_Read/PCANA(RES、AMI、MOTEC、BRAKE、STEER_SENSOR、IPC)/IPC_CMD1/IPC_Acc_Sub ==
  In1 : Inport
  Out1 : Outport
  wires:
  In1/1 -> Out1/1

== system FSAC2021_V1/VCU_CAN_Read/PCANA(RES、AMI、MOTEC、BRAKE、STEER_SENSOR、IPC)/IPC_CMD1/IPC_Brk_Sub ==
  In1 : Inport
  Out1 : Outport
  wires:
  In1/1 -> Out1/1

== system FSAC2021_V1/VCU_CAN_Read/PCANA(RES、AMI、MOTEC、BRAKE、STEER_SENSOR、IPC)/IPC_CMD1/IPC_Steer_Sub ==
  In1 : Inport
  Out1 : Outport
  wires:
  In1/1 -> Out1/1

== system FSAC2021_V1/VCU_CAN_Read/PCANA(RES、AMI、MOTEC、BRAKE、STEER_SENSOR、IPC)/Res_Message1/Res_Run_Status_Sub ==
  In1 : Inport
  Out1 : Outport
  wires:
  In1/1 -> Out1/1

== system FSAC2021_V1/VCU_CAN_Read/PCANA(RES、AMI、MOTEC、BRAKE、STEER_SENSOR、IPC)/Res_Message1/Res_check_Sub ==
  In1 : Inport
  Out1 : Outport
  wires:
  In1/1 -> Out1/1

== system FSAC2021_V1/VCU_CAN_Read/PCANA(RES、AMI、MOTEC、BRAKE、STEER_SENSOR、IPC)/Res_Message1/Safety_Relay_Sub ==
  In1 : Inport
  Out1 : Outport
  wires:
  In1/1 -> Out1/1

== system FSAC2021_V1/VCU_CAN_Read/PCANA(RES、AMI、MOTEC、BRAKE、STEER_SENSOR、IPC)/STEER_SENSOR_INFO1/Str_Sensor_Curr_Angle_Sub ==
  In1 : Inport
  Out1 : Outport
  wires:
  In1/1 -> Out1/1

== system FSAC2021_V1/VCU_CAN_Read/PCANB(BMS、DRIVE_MOTOR)/AMI_DUTY/assi_status_Sub ==
  In1 : Inport
  Out1 : Outport
  wires:
  In1/1 -> Out1/1
